simulink model "ur_mex_tester"  (R2023b)
settings: Solver=FixedStepAuto  StartTime=0.0  StopTime=80  FixedStep=0.008  RelTol=1e-3
libraries: simulink x1
settings Model: Creator=Gavin  LastModifiedBy=Gavin

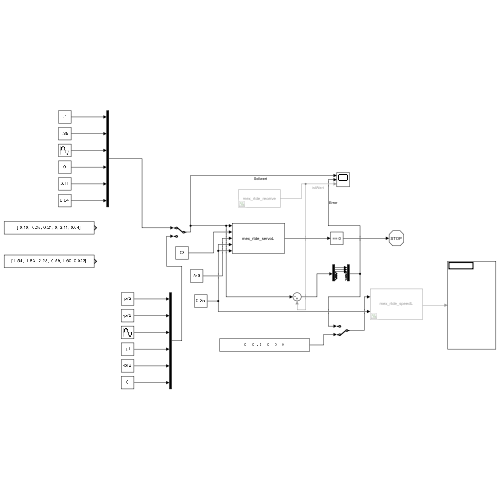
[thumbnail: Simulink's stored preview of the top-level diagram]
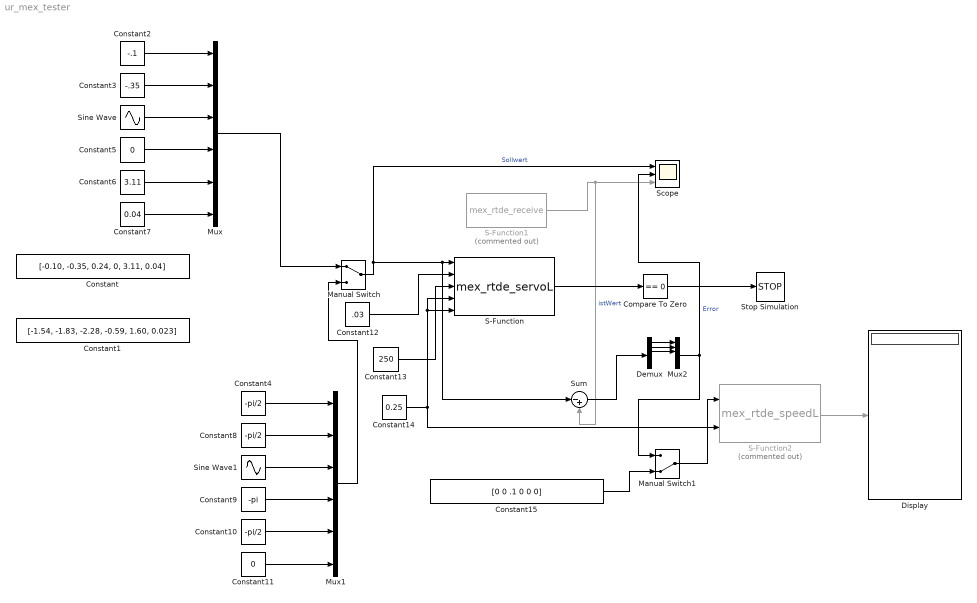
== system ur_mex_tester ==
  Compare To Zero : simulink/Logic and Bit Operations/Compare To Zero  relop===  OutDataTypeStr=boolean
  Constant : Constant  Value=[-0.10, -0.35, 0.24, 0, 3.11, 0.04]
  Constant1 : Constant  Value=[-1.54, -1.83, -2.28, -0.59, 1.60, 0.023]
  Constant10 : Constant  Value=-pi/2
  Constant11 : Constant  Value=0
  Constant12 : Constant  Value=.03
  Constant13 : Constant  Value=250
  Constant14 : Constant  Value=0.25
  Constant15 : Constant  Value=[0 0 .1 0 0 0]
  Constant2 : Constant  Value=-.1
  Constant3 : Constant  Value=-.35
  Constant4 : Constant  Value=-pi/2
  Constant5 : Constant  Value=0
  Constant6 : Constant  Value=3.11
  Constant7 : Constant  Value=0.04
  Constant8 : Constant  Value=-pi/2
  Constant9 : Constant  Value=-pi
  Demux : Demux  Outputs=6
  Display : Display
  Manual Switch : ManualSwitch
  Manual Switch1 : ManualSwitch  CurrentSetting=0
  Mux : Mux  Inputs=6
  Mux1 : Mux  Inputs=6
  Mux2 : Mux  Inputs=6
  S-Function : S-Function  FunctionName=mex_rtde_servoL  Parameters=0.008 '192.168.255.128'  SFunctionDeploymentMode=off  EnableBusSupport=off
  S-Function1 : S-Function  Commented=on  FunctionName=mex_rtde_receive  Parameters=0.008 '192.168.255.128'  SFunctionDeploymentMode=off  EnableBusSupport=off
  S-Function2 : S-Function  Commented=on  FunctionName=mex_rtde_speedL  Parameters=0.008 '192.168.255.128'  SFunctionDeploymentMode=off  EnableBusSupport=off
  Scope : Scope  NumInputPorts=3
  Sine Wave : Sin  Amplitude=0  Bias=.2  SampleTime=0.008
  Sine Wave1 : Sin  Amplitude=pi/4  Bias=pi/2  SampleTime=0.008
  Stop Simulation : Stop
  Sum : Sum  Inputs=|-+
  wires:
  Manual Switch/1 -> Scope/1, Sum/1, S-Function/1  "Sollwert"
  Constant7/1 -> Mux/6
  Constant6/1 -> Mux/5
  Constant5/1 -> Mux/4
  Constant3/1 -> Mux/2
  Constant2/1 -> Mux/1
  Sine Wave/1 -> Mux/3
  Sine Wave1/1 -> Mux1/3
  Constant4/1 -> Mux1/1
  Constant8/1 -> Mux1/2
  Constant9/1 -> Mux1/4
  Constant10/1 -> Mux1/5
  Constant11/1 -> Mux1/6
  Mux/1 -> Manual Switch/1
  Mux1/1 -> Manual Switch/2
  Constant12/1 -> S-Function/2
  Constant13/1 -> S-Function/3
  S-Function1/1 -> Scope/3, Sum/2  "istWert"
  Constant14/1 -> S-Function2/2, S-Function/5, S-Function/4
  Constant15/1 -> Manual Switch1/2
  S-Function2/1 -> Display/1
  Sum/1 -> Demux/1
  Demux/1 -> Mux2/1
  Demux/2 -> Mux2/2
  Demux/3 -> Mux2/3
  Mux2/1 -> Manual Switch1/1, Scope/2  "Error"
  Manual Switch1/1 -> S-Function2/1
  S-Function/1 -> Compare To Zero/1
  Compare To Zero/1 -> Stop Simulation/1
